simulink model "boost_close_loop"  (Simulink 10.0)
settings: Solver=ode45  StartTime=0.0  StopTime=0.04  MaxStep=0.1e-6  RelTol=1e-3  EnableMultiTasking=on
InitFcn:
  | clc;
  | clear;
  | L = 4.1e-6;
  | RL = 80e-3;
  | C = 376e-6;
  | Rc = 5e-3;
  | fs = 100e3;
  | Vg = 12;
  | D = 0.42;
  | R = 1;
StopFcn:
  | clc;
  | clear;
libraries: powerlib x17, simulink_extras x2, simulink x2
Description:
  | This model simulates two boost converter in close loop. One converts 5V to 12V while the
  | other converts 24V to 48V with the power rating of 240W.
  | 
  | This was created by
  | Syed Abdul Rahman Kashif
  | UET Lahore / UPB Germany
  | 
  | 29th April 2010
settings Model: Creator=Kashif  LastModifiedBy=bhisma
settings DataIOCC: LimitDataPoints=on  SignalLoggingSaveFormat=ModelDataLogs
settings OptimizationCC: ExpressionDepthLimit=2147483647
settings DebuggingCC: SolverPrmCheckMsg=warning  FcnCallInpInsideContextMsg=warning  StateNameClashWarn=warning
settings GRTTargetCC: GeneratePreprocessorConditionals=Disable all
settings ConfigComp: CovExternalEMLEnable=off

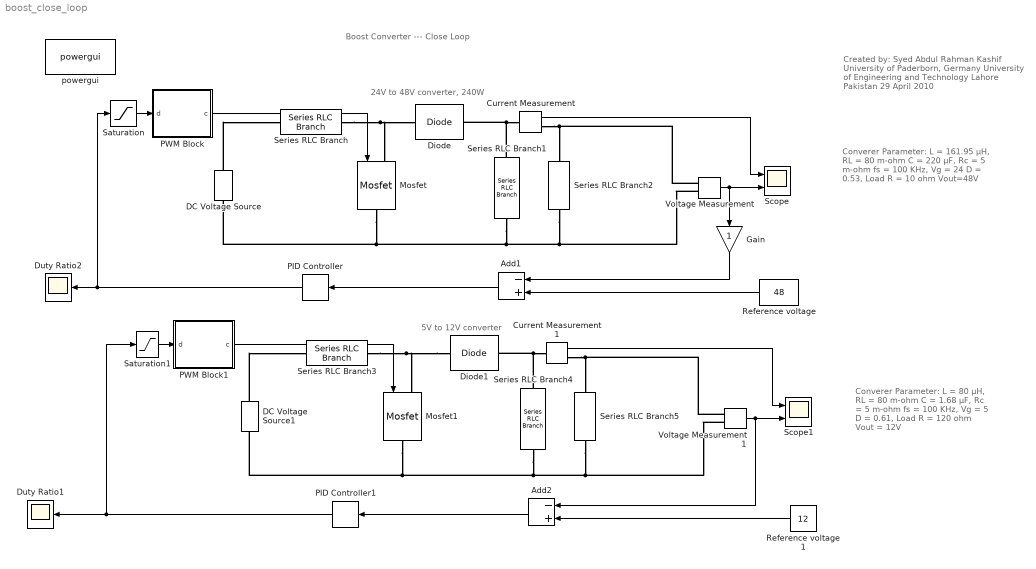
== system boost_close_loop ==
  note: Boost Converter --- Close Loop
  note: Created by: Syed Abdul Rahman Kashif
      | University of Paderborn, Germany
      | University of Engineering and Technology
      | Lahore Pakistan
      |
      | 29 April 2010
  note: Converer Parameter:
      |       L = 161.95 µH, RL = 80 m-ohm
      | C = 220 µF, Rc = 5 m-ohm
      |  	fs = 100 KHz, Vg = 24
      | D = 0.53, Load R = 10 ohm
      | Vout=48V
  note: Converer Parameter:
      |       L = 80 µH, RL = 80 m-ohm
      | C = 1.68 µF, Rc = 5 m-ohm
      |  fs = 100 KHz, Vg = 5
      | D = 0.61, Load R = 120 ohm
      | Vout = 12V
  note: 5V to 12V converter
  note: 24V to 48V converter, 240W
  Add1 : Sum  Inputs=-+
  Add2 : Sum  Inputs=-+
  Current Measurement : powerlib/Measurements/Current Measurement  SystemSampleTime=-1  PhasorSimulation=off  OutputType=Complex  PSBequivalent=0
      settings: SourceProductName=Simscape Electrical
  Current Measurement1 : powerlib/Measurements/Current Measurement  SystemSampleTime=-1  PhasorSimulation=off  OutputType=Complex  PSBequivalent=0
      settings: SourceProductName=Simscape Electrical
  DC Voltage Source : powerlib/Electrical Sources/DC Voltage Source  SystemSampleTime=-1  Amplitude=24  Measurements=None
      settings: SourceProductName=Simscape Electrical
  DC Voltage Source1 : powerlib/Electrical Sources/DC Voltage Source  SystemSampleTime=-1  Amplitude=5  Measurements=None
      settings: SourceProductName=Simscape Electrical
  Diode : powerlib/Power Electronics/Diode  SystemSampleTime=-1  Ron=0.001  Lon=0  Vf=0.8  IC=0  UseSnubber=off  Rs=500  Cs=250e-9  Measurements=off
      settings: SourceProductName=Simscape Electrical
  Diode1 : powerlib/Power Electronics/Diode  SystemSampleTime=-1  Ron=0.001  Lon=0  Vf=0.8  IC=0  UseSnubber=off  Rs=500  Cs=250e-9  Measurements=off
      settings: SourceProductName=Simscape Electrical
  Duty Ratio1 : Scope
  Duty Ratio2 : Scope
  Gain : Gain
  Mosfet : powerlib/Power Electronics/Mosfet  SystemSampleTime=-1  Ron=0.1  Lon=0  Rd=0.01  Vfd=0  IC=0  Rs=1e5  Cs=inf  Measurements=off
      settings: SourceProductName=Simscape Electrical
  Mosfet1 : powerlib/Power Electronics/Mosfet  SystemSampleTime=-1  Ron=0.1  Lon=0  Rd=0.01  Vfd=0  IC=0  Rs=1e5  Cs=inf  Measurements=off
      settings: SourceProductName=Simscape Electrical
  PID Controller : simulink_extras/Additional Linear/PID Controller  SystemSampleTime=-1  P=0  I=5  D=0
      settings: SourceProductName=Simulink  SourceProductBaseCode=SL
  PID Controller1 : simulink_extras/Additional Linear/PID Controller  SystemSampleTime=-1  P=0  I=100  D=0
      settings: SourceProductName=Simulink  SourceProductBaseCode=SL
  PWM Block : Subsystem  mask{fs=100e3}
      mask prompts: fs "Switching fFrequency"
  PWM Block1 : Subsystem  mask{fs=100e3}
      mask prompts: fs "Switching fFrequency"
  "Reference voltage " : Constant  Value=48
  Reference voltage 1 : Constant  Value=12
  Saturation : Saturate  UpperLimit=1  LowerLimit=0
  Saturation1 : Saturate  UpperLimit=1  LowerLimit=0
  Scope : Scope  NumInputPorts=2
  Scope1 : Scope  NumInputPorts=2
  Series RLC Branch : powerlib/Elements/Series RLC Branch  PhysicalDomain=powersysdomain  SubClassName=unknown  LeftPortType=p1  RightPortType=p1  LConnTagsString=__new0  RConnTagsString=__new0  BranchType=RL  Resistance=RL  Inductance=161.95e-6  SetiL0=off  InitialCurrent=0  Capacitance=1e-6  Setx0=off  InitialVoltage=0  Measurements=None
      settings: SourceProductName=Simscape Electrical
  Series RLC Branch1 : powerlib/Elements/Series RLC Branch  PhysicalDomain=powersysdomain  SubClassName=unknown  LeftPortType=p1  RightPortType=p1  LConnTagsString=__new0  RConnTagsString=__new0  BranchType=RC  Resistance=Rc  Inductance=1e-3  SetiL0=off  InitialCurrent=0  Capacitance=220e-6  Setx0=off  InitialVoltage=0  Measurements=None
      settings: SourceProductName=Simscape Electrical
  Series RLC Branch2 : powerlib/Elements/Series RLC Branch  PhysicalDomain=powersysdomain  SubClassName=unknown  LeftPortType=p1  RightPortType=p1  LConnTagsString=__new0  RConnTagsString=__new0  BranchType=R  Resistance=10  Inductance=1e-3  SetiL0=off  InitialCurrent=0  Capacitance=1e-6  Setx0=off  InitialVoltage=0  Measurements=Branch voltage and current
      settings: SourceProductName=Simscape Electrical
  Series RLC Branch3 : powerlib/Elements/Series RLC Branch  PhysicalDomain=powersysdomain  SubClassName=unknown  LeftPortType=p1  RightPortType=p1  LConnTagsString=__new0  RConnTagsString=__new0  BranchType=RL  Resistance=RL  Inductance=80e-6  SetiL0=off  InitialCurrent=0  Capacitance=1e-6  Setx0=off  InitialVoltage=0  Measurements=None
      settings: SourceProductName=Simscape Electrical
  Series RLC Branch4 : powerlib/Elements/Series RLC Branch  PhysicalDomain=powersysdomain  SubClassName=unknown  LeftPortType=p1  RightPortType=p1  LConnTagsString=__new0  RConnTagsString=__new0  BranchType=RC  Resistance=Rc  Inductance=1e-3  SetiL0=off  InitialCurrent=0  Capacitance=1.68e-6  Setx0=off  InitialVoltage=0  Measurements=None
      settings: SourceProductName=Simscape Electrical
  Series RLC Branch5 : powerlib/Elements/Series RLC Branch  PhysicalDomain=powersysdomain  SubClassName=unknown  LeftPortType=p1  RightPortType=p1  LConnTagsString=__new0  RConnTagsString=__new0  BranchType=R  Resistance=120  Inductance=1e-3  SetiL0=off  InitialCurrent=0  Capacitance=1e-6  Setx0=off  InitialVoltage=0  Measurements=Branch voltage and current
      settings: SourceProductName=Simscape Electrical
  Voltage Measurement : powerlib/Measurements/Voltage Measurement  SystemSampleTime=-1  PhasorSimulation=off  OutputType=Complex  PSBequivalent=0
      settings: SourceProductName=Simscape Electrical
  Voltage Measurement1 : powerlib/Measurements/Voltage Measurement  SystemSampleTime=-1  PhasorSimulation=off  OutputType=Complex  PSBequivalent=0
      settings: SourceProductName=Simscape Electrical
  powergui : powerlib/powergui  Priority=1  SystemSampleTime=-1  SimulationMode=Continuous  SampleTime=1e-8  frequency=60  SPID=off  DisableSnubberDevices=off  DisableRonSwitches=off  DisableVfSwitches=off  SwTol=0  Interpol=off  frequencyindice=0  echomessages=off  HookPort=off  DisplayEquations=off  FunctionMessages=off  EnableUseOfTLC=off  x0status=blocks  RestoreLinks=warning  Frange=[0:2:500]  Ylog=off  Xlog=on  ShowGrid=off  save=off  variable=ZData  structure=tpa14cfcc1_35b5_40eb_8b70_049b43167a68  ZoomFFT=off  StartTime=0.0  cycles=1  DisplayStyle=1  fundamental=60  FreqAxis=off  MaxFrequency=1000  frequencyindicesteady=1  RmsSteady=1  display=off  Ts=0  methode=off
      settings: SourceProductName=Simscape Electrical
  wires:
  PWM Block/1(c) -> Mosfet/1
  Voltage Measurement/1 -> Scope/2, Gain/1
  Current Measurement/1 -> Scope/1
  PWM Block1/1(c) -> Mosfet1/1
  Voltage Measurement1/1 -> Scope1/2, Add2/1
  Current Measurement1/1 -> Scope1/1
  PID Controller/1 -> Duty Ratio2/1, Saturation/1
  "Reference voltage "/1 -> Add1/2
  Add1/1 -> PID Controller/1
  PID Controller1/1 -> Duty Ratio1/1, Saturation1/1
  Reference voltage 1/1 -> Add2/2
  Add2/1 -> PID Controller1/1
  Saturation/1 -> PWM Block/1(d)
  Saturation1/1 -> PWM Block1/1(d)
  Gain/1 -> Add1/1
  connections:
  DC Voltage Source/RConn1 -- Series RLC Branch/LConn1
  Series RLC Branch/RConn1 -- Diode/LConn1 -- Mosfet/LConn1
  DC Voltage Source/LConn1 -- Mosfet/RConn1 -- Voltage Measurement/LConn2 -- Series RLC Branch2/RConn1 -- Series RLC Branch1/RConn1
  Voltage Measurement/LConn1 -- Series RLC Branch2/LConn1 -- Current Measurement/RConn1
  Diode/RConn1 -- Series RLC Branch1/LConn1 -- Current Measurement/LConn1
  Diode1/LConn1 -- Mosfet1/LConn1 -- Series RLC Branch3/RConn1
  Mosfet1/RConn1 -- DC Voltage Source1/LConn1 -- Series RLC Branch4/RConn1 -- Series RLC Branch5/RConn1 -- Voltage Measurement1/LConn2
  Voltage Measurement1/LConn1 -- Current Measurement1/RConn1 -- Series RLC Branch5/LConn1
  Diode1/RConn1 -- Current Measurement1/LConn1 -- Series RLC Branch4/LConn1
  DC Voltage Source1/RConn1 -- Series RLC Branch3/LConn1

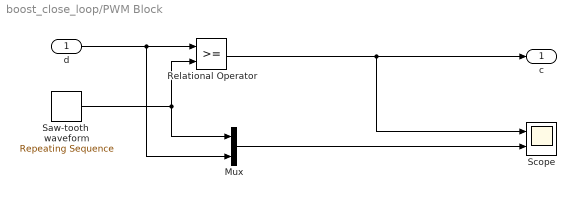
== system boost_close_loop/PWM Block ==
  d : Inport
  Mux : Mux  Inputs=2
  Relational Operator : RelationalOperator  OutDataTypeStr=boolean  RndMeth=Nearest
  Saw-tooth  waveform : simulink/Sources/Repeating Sequence  SystemSampleTime=-1  rep_seq_t=[0 1/fs]  rep_seq_y=[0 1]
  Scope : Scope  NumInputPorts=2
  c : Outport
  wires:
  d/1 -> Mux/2, Relational Operator/1
  Saw-tooth  waveform/1 -> Mux/1, Relational Operator/2
  Relational Operator/1 -> c/1, Scope/1
  Mux/1 -> Scope/2

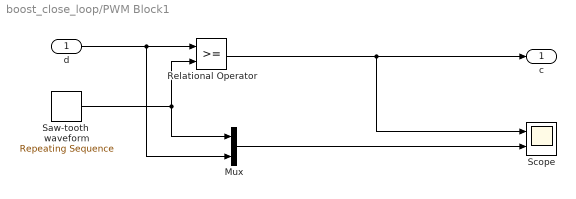
== system boost_close_loop/PWM Block1 ==
  d : Inport
  Mux : Mux  Inputs=2
  Relational Operator : RelationalOperator  OutDataTypeStr=boolean  RndMeth=Nearest
  Saw-tooth  waveform : simulink/Sources/Repeating Sequence  SystemSampleTime=-1  rep_seq_t=[0 1/fs]  rep_seq_y=[0 1]
  Scope : Scope  NumInputPorts=2
  c : Outport
  wires:
  Mux/1 -> Scope/2
  Relational Operator/1 -> Scope/1, c/1
  Saw-tooth  waveform/1 -> Relational Operator/2, Mux/1
  d/1 -> Relational Operator/1, Mux/2
